simulink model "Cruise_Simulation"  (R2018b)
settings: Solver=VariableStepAuto  StartTime=0.0  StopTime=5000  MaxStep=.1  RelTol=1e-3
values from neighbouring files (symbols this model uses):
  h0 = find_best_h(Range,Number_of_Passenger)    [main.m]
  X0 = 0    [find_best_h.m]    (also in main.m = Stations(Airplanes_Loc(counter),1))
  Xd = Range    [find_best_h.m]    (also in main.m = Stations(Next_Destination(counter),1))
  Y0 = 0    [find_best_h.m]    (also in main.m = Stations(Airplanes_Loc(counter),2))
  Yd = 0    [find_best_h.m]    (also in main.m = Stations(Next_Destination(counter),2))
undefined symbols (not defined in the file or in its folder): Alpha, CD0, CDCL, CDCL2, CL0, CLalpha, g, Gamma0, Mass, Max_RPM, Max_Tn, Number_of_Motors, Power_Compensation, Psi, S_Wing, T0, V0
libraries: aerolibatmos2 x2, simulink x1
settings Model: OrderedModelArguments=off  Creator=Arash Kiani  LastModifiedBy=User
settings DebuggingCC: AlgebraicLoopMsg=none

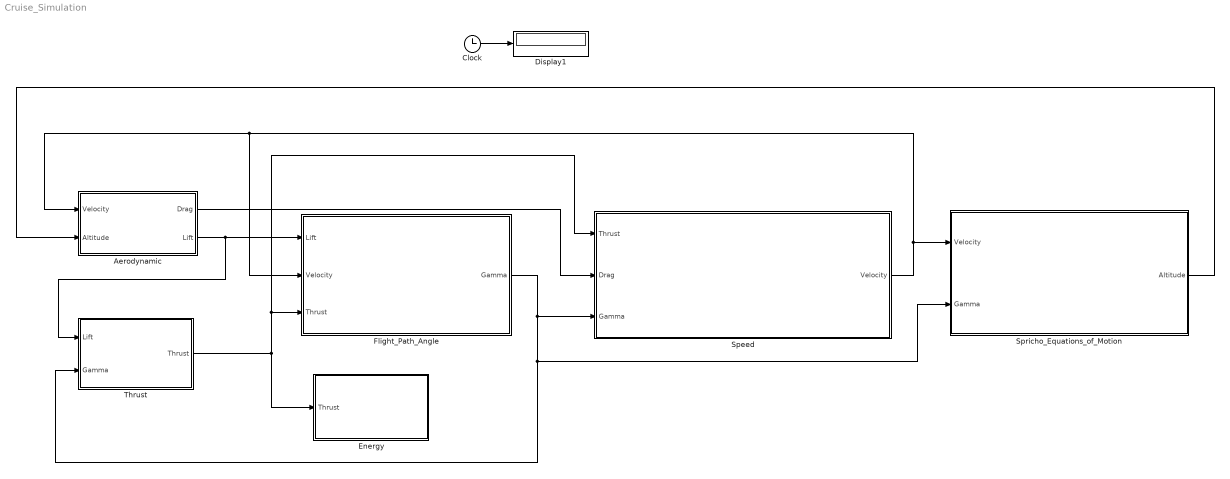
== system Cruise_Simulation ==
  "Aerodynamic " : Subsystem
  Clock : Clock
  Display1 : Display
  Energy : Subsystem
  Flight_Path_Angle : Subsystem
  Speed : Subsystem
  Spricho_Equations_of_Motion : Subsystem
  Thrust : Subsystem
  wires:
  Spricho_Equations_of_Motion/1(Altitude) -> "Aerodynamic "/2(Altitude)
  Thrust/1(Thrust) -> Energy/1("Thrust "), Flight_Path_Angle/3(Thrust), Speed/1(Thrust)
  Speed/1(Velocity) -> Spricho_Equations_of_Motion/1(Velocity), "Aerodynamic "/1(Velocity), Flight_Path_Angle/2(Velocity)
  "Aerodynamic "/2(Lift) -> Flight_Path_Angle/1(Lift), Thrust/1(Lift)
  "Aerodynamic "/1(Drag) -> Speed/2(Drag)
  Flight_Path_Angle/1(Gamma) -> Speed/3(Gamma), Spricho_Equations_of_Motion/2(Gamma), Thrust/2(Gamma)
  Clock/1 -> Display1/1

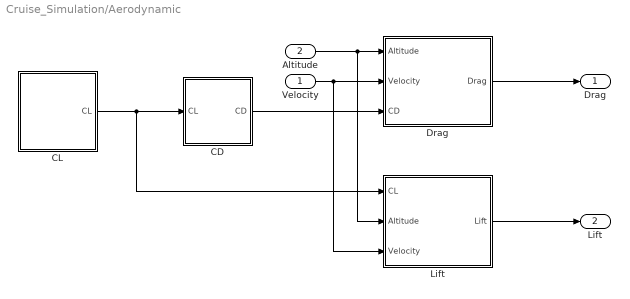
== system Cruise_Simulation/Aerodynamic  ==
  Velocity : Inport
  Altitude : Inport  Port=2
  CD : Subsystem
  CL : Subsystem
  "Drag " : Subsystem
  "Lift " : Subsystem
  Drag : Outport
  Lift : Outport  Port=2
  wires:
  "Lift "/1(Lift) -> Lift/1
  Altitude/1 -> "Lift "/2(Altitude), "Drag "/1(Altitude)
  CL/1(CL) -> CD/1(CL), "Lift "/1(CL)
  Velocity/1 -> "Lift "/3(Velocity), "Drag "/2(Velocity)
  CD/1(CD) -> "Drag "/3(CD)
  "Drag "/1(Drag) -> Drag/1

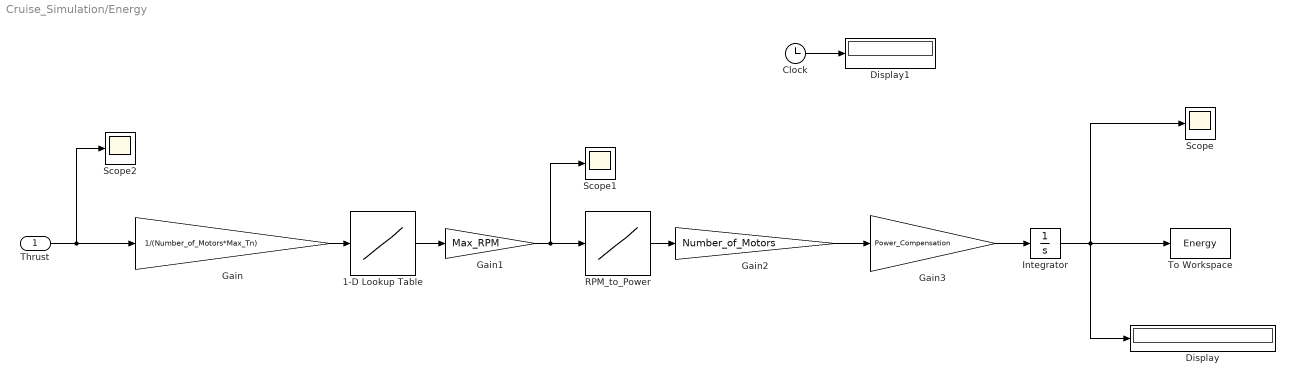
== system Cruise_Simulation/Energy ==
  "Thrust " : Inport
  1-D Lookup Table : Lookup_n-D  NumberOfTableDimensions=1  BreakpointsForDimension1=|  Table=|  InternalRulePriority=Speed  RndMeth=Simplest  InputSameDT=on
      BreakpointsForDimension1=|
      | [0	0.028414232	0.12143652	0.204120688	0.279068945	0.395219919	0.509043256	0.638242727	0.785530791	1
      | ]
      Table=|
      | [0	0.182070075	0.361369324	0.456560601	0.535171612	0.633089024	0.720012513	0.805505899	0.889658563	1
      | ]
  Clock : Clock
  Display : Display
  Display1 : Display
  Gain : Gain  Gain=1/(Number_of_Motors*Max_Tn)
  Gain1 : Gain  Gain=Max_RPM
  Gain2 : Gain  Gain=Number_of_Motors
  Gain3 : Gain  Gain=Power_Compensation
  Integrator : Integrator
  RPM_to_Power : Lookup_n-D  NumberOfTableDimensions=1  BreakpointsForDimension1=|  Table=|  InternalRulePriority=Speed  RndMeth=Simplest  InputSameDT=on
      BreakpointsForDimension1=|
      | [0	155.8	957	2115	2304	2515	2994
      | ]
      Table=|
      | [0	8078	41928	87012	95072	99855	107758
      | ]
  Scope : Scope
  Scope1 : Scope
  Scope2 : Scope
  To Workspace : ToWorkspace  VariableName=Energy  SampleTime=-1
      settings: Save2DSignal=2-D array (concatenate along first dimension)
  wires:
  Gain1/1 -> RPM_to_Power/1, Scope1/1
  "Thrust "/1 -> Gain/1, Scope2/1
  1-D Lookup Table/1 -> Gain1/1
  RPM_to_Power/1 -> Gain2/1
  Gain/1 -> 1-D Lookup Table/1
  Integrator/1 -> Display/1, To Workspace/1, Scope/1
  Gain2/1 -> Gain3/1
  Gain3/1 -> Integrator/1
  Clock/1 -> Display1/1

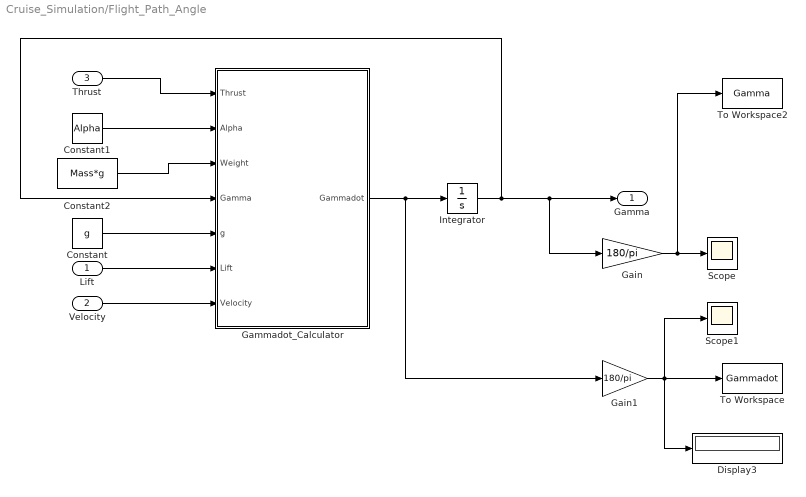
== system Cruise_Simulation/Flight_Path_Angle ==
  Lift : Inport
  Velocity : Inport  Port=2
  Thrust : Inport  Port=3
  Constant : Constant  Value=g
  Constant1 : Constant  Value=Alpha
  Constant2 : Constant  Value=Mass*g
  Display3 : Display
  Gain : Gain  Gain=180/pi
  Gain1 : Gain  Gain=180/pi
  Gammadot_Calculator : MATLAB Function  TreatAsAtomicUnit=on
  Integrator : Integrator  InitialCondition=Gamma0
  Scope : Scope
  Scope1 : Scope
  To Workspace : ToWorkspace  VariableName=Gammadot  SaveFormat=Timeseries  SampleTime=-1
      settings: Save2DSignal=2-D array (concatenate along first dimension)
  To Workspace2 : ToWorkspace  VariableName=Gamma  SaveFormat=Timeseries  SampleTime=-1
      settings: Save2DSignal=2-D array (concatenate along first dimension)
  Gamma : Outport
  wires:
  Gammadot_Calculator/1(Gammadot) -> Integrator/1, Gain1/1
  Gain1/1 -> Display3/1, Scope1/1, To Workspace/1
  Gain/1 -> To Workspace2/1, Scope/1
  Integrator/1 -> Gamma/1, Gain/1, Gammadot_Calculator/4(Gamma)
  Velocity/1 -> Gammadot_Calculator/7(Velocity)
  Lift/1 -> Gammadot_Calculator/6(Lift)
  Thrust/1 -> Gammadot_Calculator/1(Thrust)
  Constant2/1 -> Gammadot_Calculator/3(Weight)
  Constant1/1 -> Gammadot_Calculator/2(Alpha)
  Constant/1 -> Gammadot_Calculator/5(g)

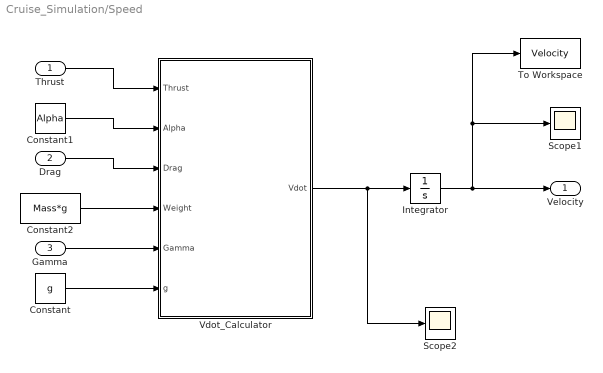
== system Cruise_Simulation/Speed ==
  Thrust : Inport
  Drag : Inport  Port=2
  Gamma : Inport  Port=3
  Constant : Constant  Value=g
  Constant1 : Constant  Value=Alpha
  Constant2 : Constant  Value=Mass*g
  Integrator : Integrator  InitialCondition=V0
  Scope1 : Scope
  Scope2 : Scope
  To Workspace : ToWorkspace  VariableName=Velocity  SaveFormat=Timeseries  SampleTime=-1
      settings: Save2DSignal=2-D array (concatenate along first dimension)
  Vdot_Calculator : MATLAB Function  TreatAsAtomicUnit=on
  Velocity : Outport
  wires:
  Vdot_Calculator/1(Vdot) -> Integrator/1, Scope2/1
  Integrator/1 -> Scope1/1, To Workspace/1, Velocity/1
  Constant/1 -> Vdot_Calculator/6(g)
  Thrust/1 -> Vdot_Calculator/1(Thrust)
  Constant1/1 -> Vdot_Calculator/2(Alpha)
  Drag/1 -> Vdot_Calculator/3(Drag)
  Gamma/1 -> Vdot_Calculator/5(Gamma)
  Constant2/1 -> Vdot_Calculator/4(Weight)

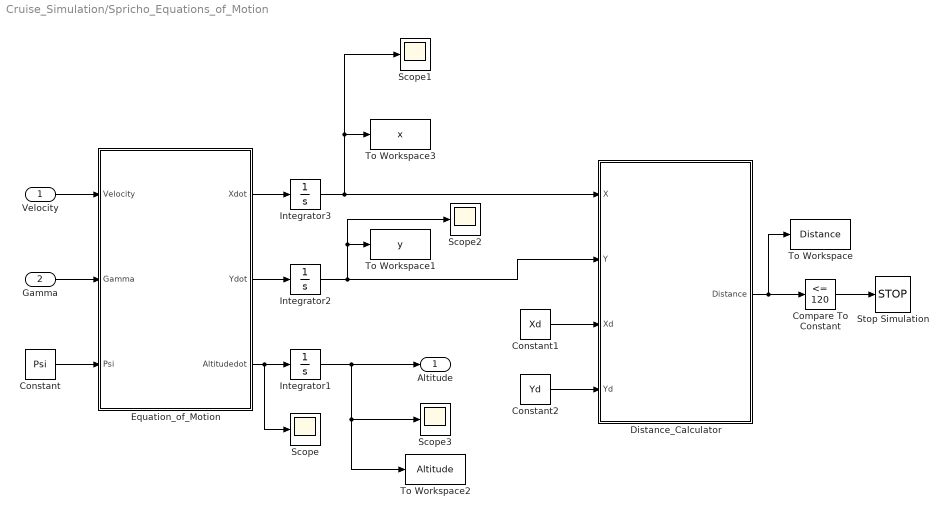
== system Cruise_Simulation/Spricho_Equations_of_Motion ==
  Velocity : Inport
  Gamma : Inport  Port=2
  Compare To Constant : simulink/Logic and Bit Operations/Compare To Constant  relop=<=  const=120  OutDataTypeStr=boolean
  Constant : Constant  Value=Psi
  Constant1 : Constant  Value=Xd
  Constant2 : Constant  Value=Yd
  Distance_Calculator : MATLAB Function  TreatAsAtomicUnit=on
  Equation_of_Motion : MATLAB Function  TreatAsAtomicUnit=on
  Integrator1 : Integrator  InitialCondition=h0
  Integrator2 : Integrator  InitialCondition=Y0
  Integrator3 : Integrator  InitialCondition=X0
  Scope{,1..3} (4 alike) : Scope
  Stop Simulation : Stop
  To Workspace : ToWorkspace  VariableName=Distance  SampleTime=-1
  To Workspace1 : ToWorkspace  VariableName=y  SampleTime=-1
  To Workspace2 : ToWorkspace  VariableName=Altitude  SampleTime=-1
      settings: Save2DSignal=2-D array (concatenate along first dimension)
  To Workspace3 : ToWorkspace  VariableName=x  SampleTime=-1
  Altitude : Outport
  wires:
  Integrator1/1 -> Scope3/1, To Workspace2/1, Altitude/1
  Integrator2/1 -> Distance_Calculator/2(Y), Scope2/1, To Workspace1/1
  Compare To Constant/1 -> Stop Simulation/1
  Velocity/1 -> Equation_of_Motion/1(Velocity)
  Gamma/1 -> Equation_of_Motion/2(Gamma)
  Constant/1 -> Equation_of_Motion/3(Psi)
  Equation_of_Motion/3(Altitudedot) -> Integrator1/1, Scope/1
  Equation_of_Motion/2(Ydot) -> Integrator2/1
  Equation_of_Motion/1(Xdot) -> Integrator3/1
  Integrator3/1 -> Scope1/1, To Workspace3/1, Distance_Calculator/1(X)
  Constant2/1 -> Distance_Calculator/4(Yd)
  Constant1/1 -> Distance_Calculator/3(Xd)
  Distance_Calculator/1(Distance) -> To Workspace/1, Compare To Constant/1

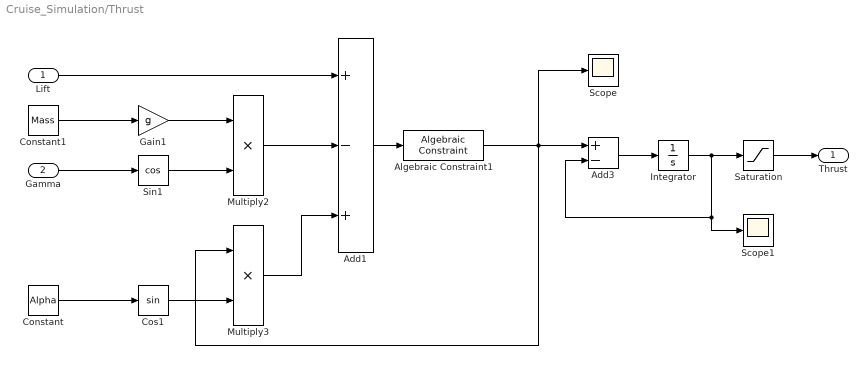
== system Cruise_Simulation/Thrust ==
  Lift : Inport
  Gamma : Inport  Port=2
  Add1 : Sum  Inputs=+-+
  Add3 : Sum  Inputs=+-
  Algebraic Constraint1 : AlgebraicConstraint
  Constant : Constant  Value=Alpha
  Constant1 : Constant  Value=Mass
  Cos1 : Trigonometry
  Gain1 : Gain  Gain=g
  Integrator : Integrator  InitialCondition=T0
  Multiply2 : Product
  Multiply3 : Product
  Saturation : Saturate  UpperLimit=inf  LowerLimit=0
  Scope : Scope
  Scope1 : Scope
  Sin1 : Trigonometry  Operator=cos
  Thrust : Outport
  wires:
  Add1/1 -> Algebraic Constraint1/1
  Cos1/1 -> Multiply3/2
  Multiply3/1 -> Add1/3
  Multiply2/1 -> Add1/2
  Constant1/1 -> Gain1/1
  Gain1/1 -> Multiply2/1
  Sin1/1 -> Multiply2/2
  Lift/1 -> Add1/1
  Constant/1 -> Cos1/1
  Gamma/1 -> Sin1/1
  Algebraic Constraint1/1 -> Add3/1, Scope/1, Multiply3/1
  Integrator/1 -> Saturation/1, Add3/2, Scope1/1
  Add3/1 -> Integrator/1
  Saturation/1 -> Thrust/1

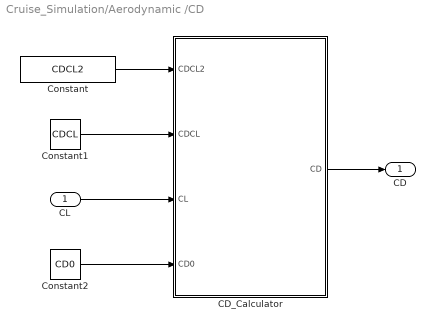
== system Cruise_Simulation/Aerodynamic /CD ==
  CL : Inport
  CD_Calculator : MATLAB Function  TreatAsAtomicUnit=on
  Constant : Constant  Value=CDCL2
  Constant1 : Constant  Value=CDCL
  Constant2 : Constant  Value=CD0
  CD : Outport
  wires:
  CL/1 -> CD_Calculator/3(CL)
  Constant/1 -> CD_Calculator/1(CDCL2)
  Constant1/1 -> CD_Calculator/2(CDCL)
  Constant2/1 -> CD_Calculator/4(CD0)
  CD_Calculator/1(CD) -> CD/1

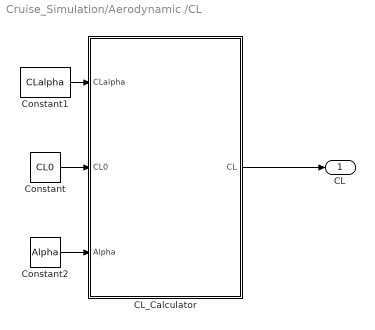
== system Cruise_Simulation/Aerodynamic /CL ==
  CL_Calculator : MATLAB Function  TreatAsAtomicUnit=on
  Constant : Constant  Value=CL0
  Constant1 : Constant  Value=CLalpha
  Constant2 : Constant  Value=Alpha
  CL : Outport
  wires:
  CL_Calculator/1(CL) -> CL/1
  Constant/1 -> CL_Calculator/2(CL0)
  Constant1/1 -> CL_Calculator/1(CLalpha)
  Constant2/1 -> CL_Calculator/3(Alpha)

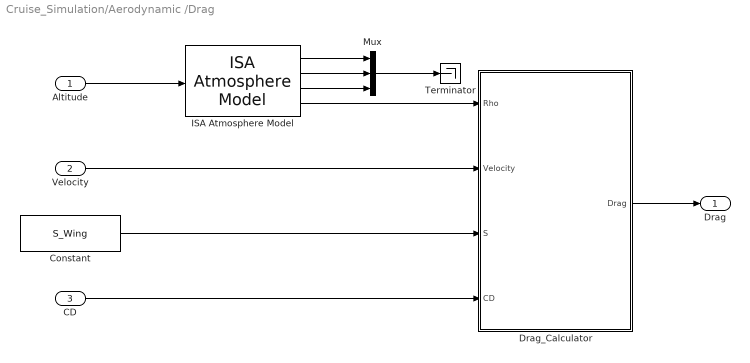
== system Cruise_Simulation/Aerodynamic /Drag  ==
  Altitude : Inport
  Velocity : Inport  Port=2
  CD : Inport  Port=3
  Constant : Constant  Value=S_Wing
  Drag_Calculator : MATLAB Function  TreatAsAtomicUnit=on
  ISA Atmosphere Model : aerolibatmos2/ISA Atmosphere Model  custom=off  g=9.80665  gamma=1.4  R=287.0531  L=0.0065  h_trop=11000  h_strat=20000  rho0=1.225  P0=101325  T0=288.15  h0=0
      settings: SourceProductName=Aerospace Blockset
  Mux : Mux  Inputs=3
  Terminator : Terminator
  Drag : Outport
  wires:
  Altitude/1 -> ISA Atmosphere Model/1
  ISA Atmosphere Model/2 -> Mux/2
  Mux/1 -> Terminator/1
  ISA Atmosphere Model/3 -> Mux/3
  ISA Atmosphere Model/1 -> Mux/1
  ISA Atmosphere Model/4 -> Drag_Calculator/1(Rho)
  Velocity/1 -> Drag_Calculator/2(Velocity)
  Constant/1 -> Drag_Calculator/3(S)
  CD/1 -> Drag_Calculator/4(CD)
  Drag_Calculator/1(Drag) -> Drag/1

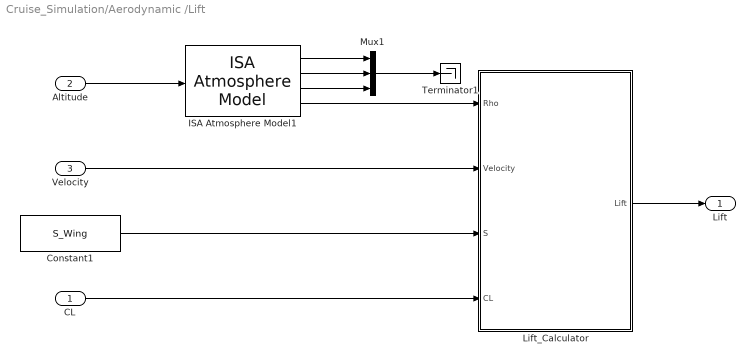
== system Cruise_Simulation/Aerodynamic /Lift  ==
  CL : Inport
  Altitude : Inport  Port=2
  Velocity : Inport  Port=3
  Constant1 : Constant  Value=S_Wing
  ISA Atmosphere Model1 : aerolibatmos2/ISA Atmosphere Model  custom=off  g=9.80665  gamma=1.4  R=287.0531  L=0.0065  h_trop=11000  h_strat=20000  rho0=1.225  P0=101325  T0=288.15  h0=0
      settings: SourceProductName=Aerospace Blockset
  Lift_Calculator : MATLAB Function  TreatAsAtomicUnit=on
  Mux1 : Mux  Inputs=3
  Terminator1 : Terminator
  Lift : Outport
  wires:
  Velocity/1 -> Lift_Calculator/2(Velocity)
  CL/1 -> Lift_Calculator/4(CL)
  Altitude/1 -> ISA Atmosphere Model1/1
  Mux1/1 -> Terminator1/1
  ISA Atmosphere Model1/3 -> Mux1/3
  ISA Atmosphere Model1/2 -> Mux1/2
  Constant1/1 -> Lift_Calculator/3(S)
  ISA Atmosphere Model1/1 -> Mux1/1
  ISA Atmosphere Model1/4 -> Lift_Calculator/1(Rho)
  Lift_Calculator/1(Lift) -> Lift/1

== matlab function Cruise_Simulation/Flight_Path_Angle/Gammadot_Calculator ==
  data: Thrust input; Gammadot output; Alpha input; Weight input; Gamma input; g input; Lift input; Velocity input
function Gammadot = fcn(Thrust,Alpha,Weight,Gamma,g,Lift,Velocity)

Gammadot = (Lift - Weight*cos(Gamma) + Thrust*sin(Alpha))*(g/(Weight*Velocity));

== matlab function Cruise_Simulation/Speed/Vdot_Calculator ==
  data: Thrust input; Vdot output; Alpha input; Drag input; Weight input; Gamma input; g input
function Vdot = fcn(Thrust,Alpha,Drag,Weight,Gamma,g)

Vdot = ((Thrust*cos(Alpha) - Drag - Weight*sin(Gamma))/Weight)*g;

== matlab function Cruise_Simulation/Aerodynamic /CD/CD_Calculator ==
  data: CDCL2 input; CD output; CDCL input; CL input; CD0 input
function CD = fcn(CDCL2,CDCL,CL,CD0)

CD = CD0 + CDCL2*(CL^2) + CDCL*CL;

== matlab function Cruise_Simulation/Aerodynamic /Drag /Drag_Calculator ==
  data: Rho input; Drag output; Velocity input; S input; CD input
function Drag = fcn(Rho,Velocity,S,CD)

Drag = 0.5*Rho*(Velocity^2)*S*CD;

== matlab function Cruise_Simulation/Aerodynamic /Lift /Lift_Calculator ==
  data: Rho input; Lift output; Velocity input; S input; CL input
function Lift = fcn(Rho,Velocity,S,CL)

Lift = 0.5*Rho*(Velocity^2)*S*CL;

== matlab function Cruise_Simulation/Spricho_Equations_of_Motion/Equation_of_Motion ==
  data: Velocity input; Gamma input; Xdot output; Psi input; Ydot output; Altitudedot output
function [Xdot,Ydot,Altitudedot] = fcn(Velocity,Gamma,Psi)

Xdot = Velocity*cos(Gamma)*cos(Psi);
Ydot = Velocity*cos(Gamma)*sin(Psi);
Altitudedot = Velocity*sin(Gamma);

== matlab function Cruise_Simulation/Spricho_Equations_of_Motion/Distance_Calculator ==
  data: X input; Y input; Distance output; Xd input; Yd input
function Distance = fcn(X,Y,Xd,Yd)

Distance = sqrt((Yd - Y)^2 + (Xd - X)^2);

== matlab function Cruise_Simulation/Aerodynamic /CL/CL_Calculator ==
  data: CLalpha input; CL output; CL0 input; Alpha input
function CL = fcn(CLalpha,CL0,Alpha)

CL = CL0 + CLalpha*Alpha;
